simulink model "rc_fir"  (Simulink 3.00)
settings: Solver=ode45  StartTime=0.0  StopTime=100000  RelTol=1e-3
undefined symbols (not defined in the file or in its folder): input_stream_sample
libraries: simulink_extras x3, dsp_blocks x2
settings Model: Creator=jon  LastModifiedBy=jon

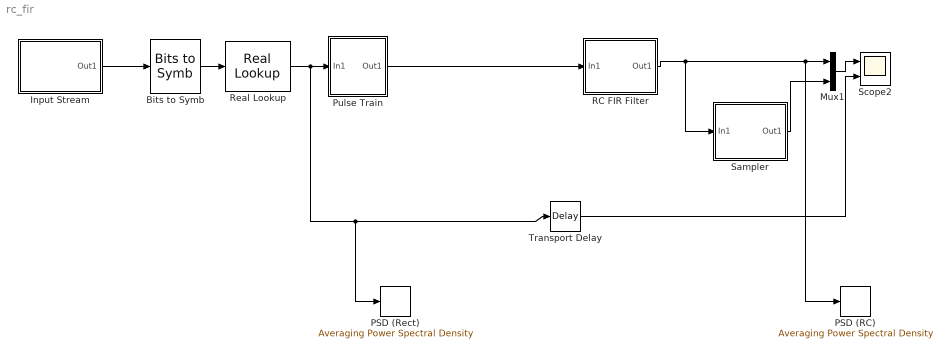
== system rc_fir ==
  Bits to Symb : dsp_blocks/Conversions/Bits to Symb
  Input Stream : Subsystem  mask{period=10, width=1, fname=rand.mat}
      mask prompts: fname "Data Filename"
      mask help: Input Stream: Reads binary data from an input file. Outputs a new value once per period. Width allows you to multiplex output.
      mask init:
      | load(fname); N = floor(length(data)/width); data = reshape(data(1:N*width),width,N);
      mask Help: The function loads the binary data from file fname, which should have a single vector called "data".  The output of the block is updated once every T=width*period.
      mask Display: disp(sprintf('file=%s\nT=%g w=%d', fname, period, width))
  Mux1 : Mux  Inputs=2
  PSD (RC) : simulink_extras/Additional Sinks/Averaging Power Spectral Density  npts=16384  fftpts=256  HowOften=2048  sampleT=1
  PSD (Rect) : simulink_extras/Additional Sinks/Averaging Power Spectral Density  npts=16384  fftpts=256  HowOften=2048  sampleT=1
  Pulse Train : Subsystem  mask{period=10}
      mask prompts: period "Period (samples)"
      mask help: Samples the incoming signal and makes a pulse train.
      mask Display: disp(sprintf('T=%d', period));
  RC FIR Filter : Subsystem  mask{period=10, beta=0.5, root=off, filt_len=128}
      mask prompts: period "Symbol Period"; beta "Roll Off (beta)"; root "Root Filter?"; filt_len "Filter Length (taps)"
      mask init:
      | symb_rate = 1/period; p.fs = symb_rate; p.beta = beta; p.root = root; [h f Ha Hi win] = win_method('rc_filt', p, 0.5, 1, filt_len, 1); h = h';
      mask Display: plot(f, abs(Ha));
  Real Lookup : dsp_blocks/Conversions/Real Lookup  table=[-1 1]
  Sampler : Subsystem  mask{offset=64, samp_period=10}
      mask prompts: offset "Offset (samples)"; samp_period "Sample Period"
      mask Display: disp(sprintf('del=%d, T=%d', offset, samp_period));
  Scope2 : Scope  NumInputPorts=2
      settings: TimeRange=auto  YMin=-5~-5  YMax=5~5  SaveToWorkspace=off  SaveName=ScopeData  LimitMaxRows=off
  Transport Delay : TransportDelay  DelayTime=64  InitialInput=1  BufferSize=1024
  wires:
  Input Stream/1(Out1) -> Bits to Symb/1
  Bits to Symb/1 -> Real Lookup/1
  RC FIR Filter/1(Out1) -> Sampler/1(In1), Mux1/1, PSD (RC)/1
  Mux1/1 -> Scope2/1
  Sampler/1(Out1) -> Mux1/2
  Real Lookup/1 -> Pulse Train/1(In1), Transport Delay/1, PSD (Rect)/1
  Pulse Train/1(Out1) -> RC FIR Filter/1(In1)
  Transport Delay/1 -> Scope2/2

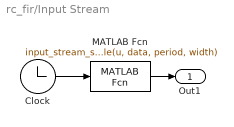
== system rc_fir/Input Stream ==
  Clock : Clock
  MATLAB Fcn : MATLABFcn  MATLABFcn=input_stream_sample(u, data, period, width)  OutputWidth=width  OutputSignalType=auto
  Out1 : Outport  Port=1
  wires:
  MATLAB Fcn/1 -> Out1/1
  Clock/1 -> MATLAB Fcn/1

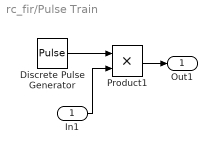
== system rc_fir/Pulse Train ==
  In1 : Inport  Port=1  PortWidth=-1  SampleTime=-1  DataType=auto
      settings: SignalType=auto
  Discrete Pulse Generator : DiscretePulseGenerator  Amplitude=1  Period=period  PulseWidth=1  PhaseDelay=0  SampleTime=1
  Product1 : Product  Inputs=2  SaturateOnIntegerOverflow=on
  Out1 : Outport  Port=1
  wires:
  Discrete Pulse Generator/1 -> Product1/1
  Product1/1 -> Out1/1
  In1/1 -> Product1/2

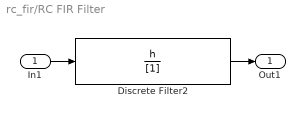
== system rc_fir/RC FIR Filter ==
  In1 : Inport  Port=1  PortWidth=-1  SampleTime=-1  DataType=auto
      settings: SignalType=auto
  Discrete Filter2 : DiscreteFilter  Numerator=h  Denominator=[1]  SampleTime=1
  Out1 : Outport  Port=1
  wires:
  In1/1 -> Discrete Filter2/1
  Discrete Filter2/1 -> Out1/1

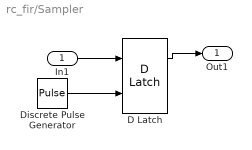
== system rc_fir/Sampler ==
  In1 : Inport  Port=1  PortWidth=-1  SampleTime=-1  DataType=auto
      settings: SignalType=auto
  D Latch : simulink_extras/Flip Flops/D Latch
  Discrete Pulse Generator : DiscretePulseGenerator  Amplitude=1  Period=samp_period  PulseWidth=1  PhaseDelay=offset  SampleTime=1
  Out1 : Outport  Port=1
  wires:
  Discrete Pulse Generator/1 -> D Latch/2
  In1/1 -> D Latch/1
  D Latch/1 -> Out1/1
